simulink model "Golf_Nonlin_Final"  (R2019a)
settings: Solver=ode45  StartTime=0.0  StopTime=400  MaxStep=1.2  RelTol=1e-3
values from neighbouring files (symbols this model uses):
  A6 = Acm(iVa:end, iVa:end)    [mainProjetCADV_2a.m]
  alphaTrim = trimVal(2)    [mainProjetCADV_2a.m]
  alphaTrimLF = trimValLF(2)    [mainProjetCADV_2a.m]
  Ar = [-3/taero, 0 ... (first row only)    [mainProjetCADV_2a.m]
  B6 = Bcm(iVa:end)    [mainProjetCADV_2a.m]
  Br = [3/taero, 0 ... (first row only)    [mainProjetCADV_2a.m]
  Cobs = [C6(1,:); C6(3,:); C6(4,:)]    [mainProjetCADV_2a.m]
  DEG2RAD = pi/180.    (= 0.0174532925199)    [mainProjetCADV_2a.m]    (also in utAcDynamicsFunction.m; utConstantAeroCoeff.m)
  Dpf = K_aug * [Nx; Nxr] + Nu    [mainProjetCADV_2a.m]
  dPHRTrim = trimVal(1)    [mainProjetCADV_2a.m]
  dPHRTrimLF = trimValLF(1)    [mainProjetCADV_2a.m]
  dthrIdle = 0.1    [mainProjetCADV_2a.m]
  dthrTrimLF = trimValLF(3)    [mainProjetCADV_2a.m]
  FL2M = 30.48    [mainProjetCADV_2a.m]    (also in utAcDynamicsFunction.m)
  K_i = K_aug(end)    [mainProjetCADV_2a.m]
  K_x = K_aug(1:end-1)    [mainProjetCADV_2a.m]
  km = trim.kmass(choix)    [utGetTrimPoint.m]
  Kr = K_aug(:, 5:6)    [mainProjetCADV_2a.m]
  KTS2MS = 1852 / 3600    (= 0.514444444444)    [mainProjetCADV_2a.m]    (also in utAcDynamicsFunction.m)
  Kx = K_aug(:, 1:4)    [mainProjetCADV_2a.m]
  L6 = L6t'    [mainProjetCADV_2a.m]
  ms = trim.mStat(choix)    [utGetTrimPoint.m]
  thetaTrim = trimVal(3)    [mainProjetCADV_2a.m]
  thetaTrimLF = trimValLF(2)    [mainProjetCADV_2a.m]
  uTrim = zeros(TOTAL_CMD, 1)    [mainProjetCADV_2a.m]
  VaTrim = utEas2Tas(Eas_KTS*KTS2MS, hTrimFL*FL2M)    [mainProjetCADV_2a.m]
  VaTrimLF = utEas2Tas(230*KTS2MS, hTrimLF)    [mainProjetCADV_2a.m]
  xTrim = zeros(TOTAL_SV, 1)    [mainProjetCADV_2a.m]
undefined symbols (not defined in the file or in its folder): aircraftChosen, Eas_KTS, Kd, Ki, Kp
settings Model: Creator=mariu  LastModifiedBy=ulyss

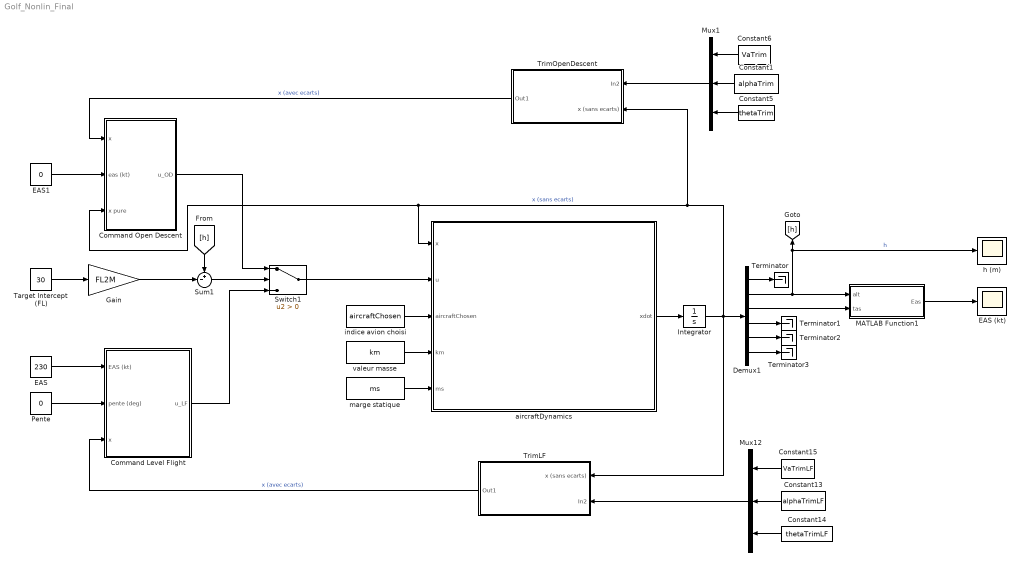
== system Golf_Nonlin_Final ==
  Command Level Flight : Subsystem
  Command Open Descent : Subsystem
  Constant1 : Constant  Value=alphaTrim
  Constant13 : Constant  Value=alphaTrimLF
  Constant14 : Constant  Value=thetaTrimLF
  Constant15 : Constant  Value=VaTrimLF
  Constant5 : Constant  Value=thetaTrim
  Constant6 : Constant  Value=VaTrim
  Demux1 : Demux  Outputs=6
  EAS : Constant  Value=230
  EAS (kt) : Scope
  EAS1 : Constant  Value=0
  Gain : Gain  Gain=FL2M
  Integrator : Integrator  InitialCondition=xTrim
  MATLAB Function1 : MATLAB Function  TreatAsAtomicUnit=on
  Mux1 : Mux  Inputs=3
  Mux12 : Mux  Inputs=3
  Pente : Constant  Value=0
  Sum1 : Sum  Inputs=+-|
  Switch1 : Switch  Criteria=u2 > Threshold
  Target Intercept (FL) : Constant  Value=30
  Terminator{,1..3} (4 alike) : Terminator
  TrimLF : Subsystem
  TrimOpenDescent : Subsystem
  aircraftDynamics : MATLAB Function  TreatAsAtomicUnit=on
  h (m) : Scope
  indice avion choisi : Constant  Value=aircraftChosen
  marge statique : Constant  Value=ms
  valeur masse : Constant  Value=km
  wires:
  aircraftDynamics/1(xdot) -> Integrator/1
  indice avion choisi/1 -> aircraftDynamics/3(aircraftChosen)
  marge statique/1 -> aircraftDynamics/5(ms)
  valeur masse/1 -> aircraftDynamics/4(km)
  MATLAB Function1/1(Eas) -> EAS (kt)/1
  EAS/1 -> Command Level Flight/1(EAS (kt))
  Pente/1 -> Command Level Flight/2(pente (deg))
  EAS1/1 -> Command Open Descent/2(eas (kt))
  Target Intercept (FL)/1 -> Gain/1
  Sum1/1 -> Switch1/2
  Gain/1 -> Sum1/2
  Constant14/1 -> Mux12/3
  Constant13/1 -> Mux12/2
  Constant15/1 -> Mux12/1
  Demux1/3 -> MATLAB Function1/2(tas)
  Demux1/2 -> MATLAB Function1/1(alt), h (m)/1, [h]  "h"
  Demux1/4 -> Terminator1/1
  Demux1/5 -> Terminator2/1
  Demux1/1 -> Terminator/1
  Demux1/6 -> Terminator3/1
  Mux12/1 -> TrimLF/2(In2)
  TrimLF/1(Out1) -> Command Level Flight/3(x)  "x (avec ecarts)"
  Integrator/1 -> TrimLF/1(x (sans ecarts)), Demux1/1, TrimOpenDescent/2(x (sans ecarts)), Command Open Descent/3(x pure), aircraftDynamics/1(x)  "x (sans ecarts)"
  Mux1/1 -> TrimOpenDescent/1(In2)
  Constant5/1 -> Mux1/3
  Constant1/1 -> Mux1/2
  Constant6/1 -> Mux1/1
  TrimOpenDescent/1(Out1) -> Command Open Descent/1(x)  "x (avec ecarts)"
  [h] -> Sum1/1
  Switch1/1 -> aircraftDynamics/2(u)
  Command Open Descent/1(u_OD) -> Switch1/1
  Command Level Flight/1(u_LF) -> Switch1/3

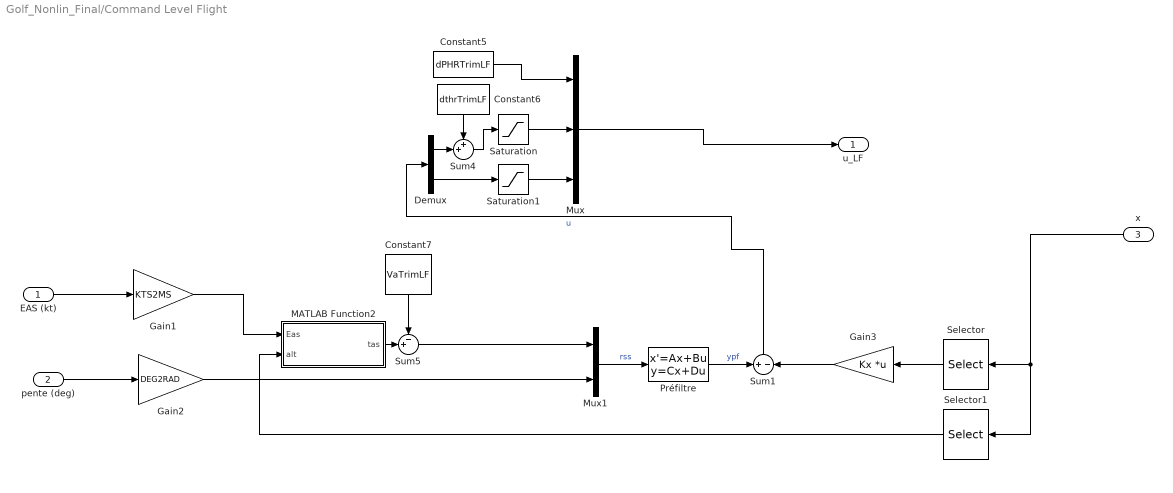
== system Golf_Nonlin_Final/Command Level Flight ==
  EAS (kt) : Inport
  pente (deg) : Inport  Port=2
  x : Inport  Port=3
  Constant5 : Constant  Value=dPHRTrimLF
  Constant6 : Constant  Value=dthrTrimLF
  Constant7 : Constant  Value=VaTrimLF
  Demux : Demux  Outputs=2
  Gain1 : Gain  Gain=KTS2MS
  Gain2 : Gain  Gain=DEG2RAD
  Gain3 : Gain  Gain=Kx  Multiplication=Matrix(K*u) (u vector)
  MATLAB Function2 : MATLAB Function  TreatAsAtomicUnit=on
  Mux : Mux  Inputs=3
  Mux1 : Mux  Inputs=2
  Préfiltre : StateSpace  A=Ar  B=Br  C=-Kr  D=Dpf  InitialCondition=0
  Saturation : Saturate  UpperLimit=1  LowerLimit=0
  Saturation1 : Saturate  UpperLimit=35*DEG2RAD  LowerLimit=-35*DEG2RAD
  Selector : Selector  InputPortWidth=6  IndexOptions=Index vector (dialog)  Indices=[3:6]  OutputSizes=1
  Selector1 : Selector  InputPortWidth=6  IndexOptions=Index vector (dialog)  Indices=[2]  OutputSizes=1
  Sum1 : Sum  Inputs=+|-
  Sum4 : Sum  Inputs=++|
  Sum5 : Sum  Inputs=-+|
  u_LF : Outport
  wires:
  Sum1/1 -> Demux/1  "u"
  Constant5/1 -> Mux/1
  Mux/1 -> u_LF/1
  Demux/1 -> Sum4/2
  Demux/2 -> Saturation1/1
  Sum4/1 -> Saturation/1
  Mux1/1 -> Préfiltre/1  "rss"
  Constant6/1 -> Sum4/1
  Saturation/1 -> Mux/2
  Gain2/1 -> Mux1/2
  MATLAB Function2/1(tas) -> Sum5/2
  Gain3/1 -> Sum1/2
  Sum5/1 -> Mux1/1
  Gain1/1 -> MATLAB Function2/1(Eas)
  Préfiltre/1 -> Sum1/1  "ypf"
  Constant7/1 -> Sum5/1
  Selector/1 -> Gain3/1
  Saturation1/1 -> Mux/3
  pente (deg)/1 -> Gain2/1
  EAS (kt)/1 -> Gain1/1
  x/1 -> Selector1/1, Selector/1
  Selector1/1 -> MATLAB Function2/2(alt)

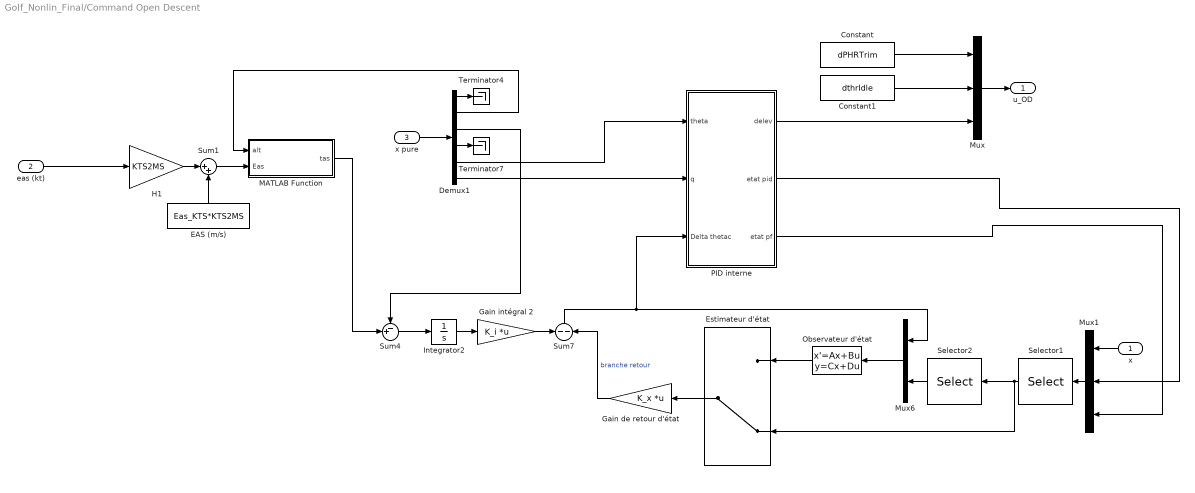
== system Golf_Nonlin_Final/Command Open Descent ==
  x : Inport
  eas (kt) : Inport  Port=2
  x pure : Inport  Port=3
  Constant : Constant  Value=dPHRTrim
  Constant1 : Constant  Value=dthrIdle
  Demux1 : Demux  Outputs=6
  EAS (m/s) : Constant  Value=Eas_KTS*KTS2MS
  Estimateur d'état : ManualSwitch  CurrentSetting=0
  Gain de retour d'état : Gain  Gain=K_x  Multiplication=Matrix(K*u) (u vector)
  Gain intégral 2 : Gain  Gain=K_i  Multiplication=Matrix(K*u) (u vector)
  H1 : Gain  Gain=KTS2MS
  Integrator2 : Integrator
  MATLAB Function : MATLAB Function  TreatAsAtomicUnit=on
  Mux : Mux  Inputs=3
  Mux1 : Mux  Inputs=3
  Mux6 : Mux  Inputs=2
  Observateur d'état : StateSpace  A=A6-L6*Cobs  B=[B6, L6]  C=eye(6)  D=zeros(6,4)  InitialCondition=0
  PID interne : Subsystem
  Selector1 : Selector  InputPortWidth=8  IndexOptions=Index vector (dialog)  Indices=[3:8]  OutputSizes=1
  Selector2 : Selector  InputPortWidth=6  IndexOptions=Index vector (dialog)  Indices=[1,3,4]  OutputSizes=1
  Sum1 : Sum  Inputs=|++
  Sum4 : Sum  Inputs=-+|
  Sum7 : Sum  Inputs=-|-
  Terminator4 : Terminator
  Terminator7 : Terminator
  u_OD : Outport
  wires:
  H1/1 -> Sum1/1
  Mux6/1 -> Observateur d'état/1
  Integrator2/1 -> Gain intégral 2/1
  Gain de retour d'état/1 -> Sum7/2  "branche retour"
  Gain intégral 2/1 -> Sum7/1
  Estimateur d'état/1 -> Gain de retour d'état/1
  Sum4/1 -> Integrator2/1
  MATLAB Function/1(tas) -> Sum4/2
  Observateur d'état/1 -> Estimateur d'état/1
  EAS (m/s)/1 -> Sum1/2
  eas (kt)/1 -> H1/1
  Mux/1 -> u_OD/1
  Constant/1 -> Mux/1
  Constant1/1 -> Mux/2
  Selector2/1 -> Mux6/2
  Demux1/3 -> Sum4/1
  Sum7/1 -> PID interne/3("Delta thetac "), Mux6/1
  PID interne/1(delev) -> Mux/3
  x pure/1 -> Demux1/1
  Demux1/6 -> PID interne/2(q)
  Demux1/5 -> PID interne/1(theta)
  Demux1/1 -> Terminator4/1
  Demux1/2 -> MATLAB Function/1(alt)
  Demux1/4 -> Terminator7/1
  Sum1/1 -> MATLAB Function/2(Eas)
  PID interne/2(etat pid) -> Mux1/2
  PID interne/3("etat pf ") -> Mux1/3
  x/1 -> Mux1/1
  Selector1/1 -> Estimateur d'état/2, Selector2/1
  Mux1/1 -> Selector1/1

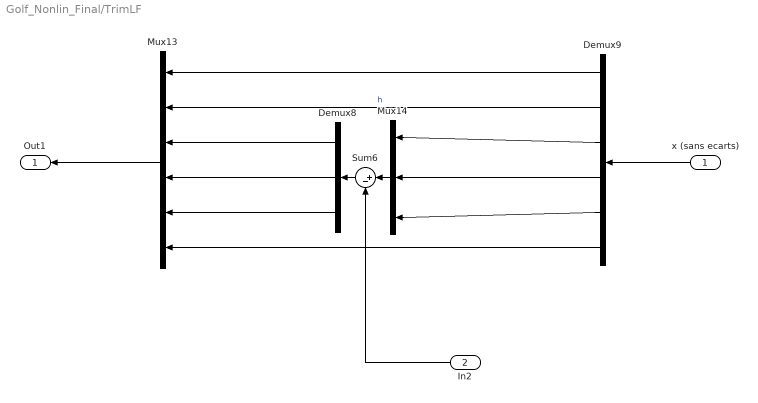
== system Golf_Nonlin_Final/TrimLF ==
  x (sans ecarts) : Inport
  In2 : Inport  Port=2
  Demux8 : Demux  Outputs=3
  Demux9 : Demux  Outputs=6
  Mux13 : Mux  Inputs=6
  Mux14 : Mux  Inputs=3
  Sum6 : Sum  Inputs=|+-
  Out1 : Outport
  wires:
  Sum6/1 -> Demux8/1
  Demux9/6 -> Mux13/6
  Demux9/4 -> Mux14/2
  Demux9/5 -> Mux14/3
  Demux8/2 -> Mux13/4
  Demux8/3 -> Mux13/5
  Demux9/3 -> Mux14/1
  Demux8/1 -> Mux13/3
  Demux9/2 -> Mux13/2  "h"
  Demux9/1 -> Mux13/1
  Mux14/1 -> Sum6/1
  x (sans ecarts)/1 -> Demux9/1
  Mux13/1 -> Out1/1
  In2/1 -> Sum6/2

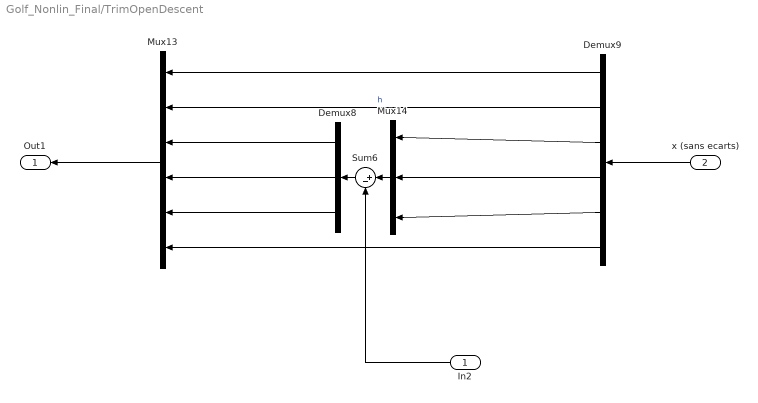
== system Golf_Nonlin_Final/TrimOpenDescent ==
  In2 : Inport
  x (sans ecarts) : Inport  Port=2
  Demux8 : Demux  Outputs=3
  Demux9 : Demux  Outputs=6
  Mux13 : Mux  Inputs=6
  Mux14 : Mux  Inputs=3
  Sum6 : Sum  Inputs=|+-
  Out1 : Outport
  wires:
  Sum6/1 -> Demux8/1
  Demux9/6 -> Mux13/6
  Demux9/4 -> Mux14/2
  Demux9/5 -> Mux14/3
  Demux8/2 -> Mux13/4
  Demux8/3 -> Mux13/5
  Demux9/3 -> Mux14/1
  Demux8/1 -> Mux13/3
  Demux9/2 -> Mux13/2  "h"
  Demux9/1 -> Mux13/1
  Mux14/1 -> Sum6/1
  x (sans ecarts)/1 -> Demux9/1
  Mux13/1 -> Out1/1
  In2/1 -> Sum6/2

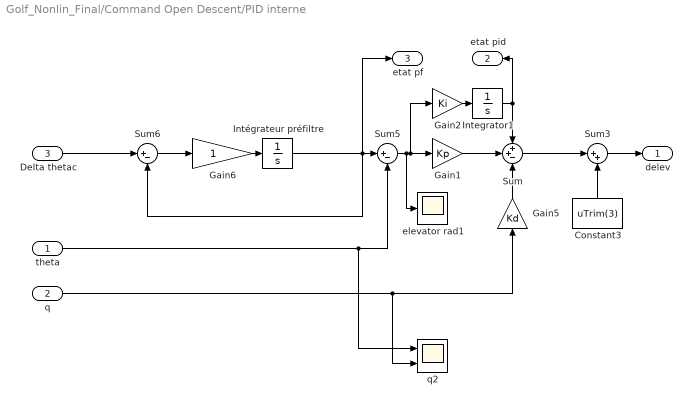
== system Golf_Nonlin_Final/Command Open Descent/PID interne ==
  theta : Inport
  q : Inport  Port=2
  "Delta thetac " : Inport  Port=3
  Constant3 : Constant  Value=uTrim(3)
  Gain1 : Gain  Gain=Kp
  Gain2 : Gain  Gain=Ki
  Gain5 : Gain  Gain=Kd
  Gain6 : Gain
  Integrator1 : Integrator
  Intégrateur préfiltre : Integrator
  Sum : Sum  Inputs=++-
  Sum3 : Sum  Inputs=|++
  Sum5 : Sum  Inputs=|+-
  Sum6 : Sum  Inputs=|+-
  elevator rad1 : Scope
  q2 : Scope  NumInputPorts=2
  delev : Outport
  etat pid : Outport  Port=2
  "etat pf " : Outport  Port=3
  wires:
  Gain2/1 -> Integrator1/1
  Sum/1 -> Sum3/1
  Sum5/1 -> elevator rad1/1, Gain2/1, Gain1/1
  Integrator1/1 -> etat pid/1, Sum/1
  Gain5/1 -> Sum/3
  Intégrateur préfiltre/1 -> "etat pf "/1, Sum6/2, Sum5/1
  Gain1/1 -> Sum/2
  "Delta thetac "/1 -> Sum6/1
  Sum6/1 -> Gain6/1
  Constant3/1 -> Sum3/2
  q/1 -> q2/2, Gain5/1
  Gain6/1 -> Intégrateur préfiltre/1
  Sum3/1 -> delev/1
  theta/1 -> q2/1, Sum5/2

== matlab function Golf_Nonlin_Final/Command Level Flight/MATLAB Function2 ==
  data: Eas input; alt input; tas output
function tas = utEas2tas(Eas, alt)
    %tas, Eas (%equivalent vitesse) en m/s
    %alt en m
    %cf. http://www.hochwarth.com/misc/AviationCalculator.html
    tas = sqrt(utRho(0)/utRho(alt))*Eas;
end

== matlab function Golf_Nonlin_Final/aircraftDynamics ==
  data: x input; u input; xdot output; aircraftChosen input; km input; ms input
function xdot = aircraftDynamics(x,u, aircraftChosen,km,ms)
    TOTAL_SV = 6;
    xIn = zeros(TOTAL_SV,1);
    xIn = x;
    
	TOTAL_CMD = 3;
    uIn = zeros(TOTAL_CMD,1);
    uIn = u;
    
    xdot = utAcDynamicsFunction(xIn,uIn, aircraftChosen,km,ms);
end %aircraftDynamics

== matlab function Golf_Nonlin_Final/MATLAB Function1 ==
  data: alt input; tas input; Eas output
function Eas = utTas2Eas(alt, tas)
    %tas, Eas(%equivalent vitesse) en m/s
    %alt en m
    %cf. http://www.hochwarth.com/misc/AviationCalculator.html
    Eas = sqrt(utRho(alt)/utRho(0))*tas/0.5144;
    %sortie en kt
end

== matlab function Golf_Nonlin_Final/Command Open Descent/MATLAB Function ==
  data: alt input; Eas input; tas output
function tas = utEas2tas(alt, Eas)
    %tas, Eas (%equivalent vitesse) en m/s
    %alt en m
    %cf. http://www.hochwarth.com/misc/AviationCalculator.html
    tas = sqrt(utRho(0)/utRho(alt))*Eas;
end
